simulink model "am"  (R2013b)
settings: Solver=ode45  StartTime=0.0  StopTime=10.0  RelTol=1e-3
undefined symbols (not defined in the file): fdesignblkfcn, gcbh
libraries: dspsrcs4 x1
settings Model: Creator=Nouri  LastModifiedBy=Ali

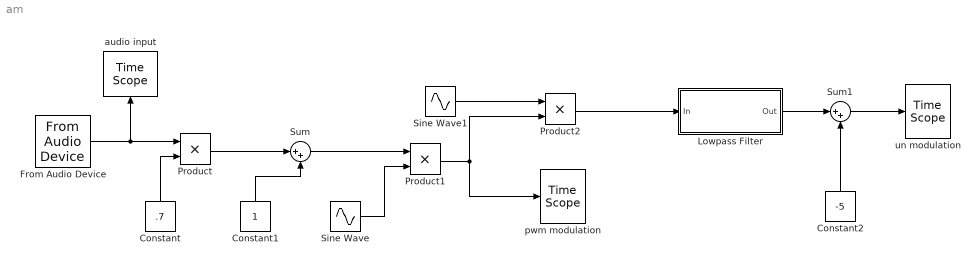
== system am ==
  Constant : Constant  Value=.7  OutDataTypeStr=single
  Constant1 : Constant  OutDataTypeStr=single
  Constant2 : Constant  Value=-5  OutDataTypeStr=single
  From Audio Device : dspsrcs4/From Audio Device  deviceName=Default  numChannels=1  sampleRate=1200  deviceDatatype=Determine from output data type  autoBufferSize=on  bufferSize=4096  queueDuration=5  frameSize=1  outputDatatype=single  defaultInputChannelMapping=on  inputChannelMapping=1:2
  Lowpass Filter : Subsystem  DialogController=fdesignblkfcn  InitFcn=fdesignblkfcn(gcbh, {'InitFcn'});  mask(Lowpass Filter){}
      mask help: Design a lowpass filter
      settings: CopyFcn=fdesignblkfcn(gcbh, {'CopyFcn'});
      mask Help: helpview(mapfilelocation('dsp'), 'dsplowpassfilter');
      mask Display: disp('Lowpass')
  Product : Product
  Product1 : Product
  Product2 : Product
  Sine Wave : Sin  Amplitude=2  Frequency=20000  SampleTime=0
  Sine Wave1 : Sin  Amplitude=2  Frequency=20000  SampleTime=0
  Sum : Sum  Inputs=|++
  Sum1 : Sum  Inputs=|++
  audio input : TimeScope  DefaultConfigurationName=spbscopes.TimeScopeBlockCfg
      settings: CopyFcn=scopeextensions.ScopeBlock.onCoreBlockCopy(gcbh);  DeleteFcn=scopeextensions.ScopeBlock.callback(gcbh, 'onBlockDelete');  PreSaveFcn=scopeextensions.ScopeBlock.callback(gcbh, 'onModelSave');  NameChangeFcn=scopeextensions.ScopeBlock.callback(gcbh, 'onBlockRename');  DestroyFcn=scopeextensions.ScopeBlock.onBlockDestroy(gcbh)  CloseFcn=scopeextensions.ScopeBlock.callback(gcbh, 'onBlockClose');  PreDeleteFcn=scopeextensions.ScopeBlock.callback(gcbh, 'onBlockPreDelete');
  pwm modulation : TimeScope  DefaultConfigurationName=spbscopes.TimeScopeBlockCfg
      settings: CopyFcn=scopeextensions.ScopeBlock.onCoreBlockCopy(gcbh);  DeleteFcn=scopeextensions.ScopeBlock.callback(gcbh, 'onBlockDelete');  PreSaveFcn=scopeextensions.ScopeBlock.callback(gcbh, 'onModelSave');  NameChangeFcn=scopeextensions.ScopeBlock.callback(gcbh, 'onBlockRename');  DestroyFcn=scopeextensions.ScopeBlock.onBlockDestroy(gcbh)  CloseFcn=scopeextensions.ScopeBlock.callback(gcbh, 'onBlockClose');  PreDeleteFcn=scopeextensions.ScopeBlock.callback(gcbh, 'onBlockPreDelete');
  un modulation : TimeScope  DefaultConfigurationName=spbscopes.TimeScopeBlockCfg
      settings: CopyFcn=scopeextensions.ScopeBlock.onCoreBlockCopy(gcbh);  DeleteFcn=scopeextensions.ScopeBlock.callback(gcbh, 'onBlockDelete');  PreSaveFcn=scopeextensions.ScopeBlock.callback(gcbh, 'onModelSave');  NameChangeFcn=scopeextensions.ScopeBlock.callback(gcbh, 'onBlockRename');  DestroyFcn=scopeextensions.ScopeBlock.onBlockDestroy(gcbh)  CloseFcn=scopeextensions.ScopeBlock.callback(gcbh, 'onBlockClose');  PreDeleteFcn=scopeextensions.ScopeBlock.callback(gcbh, 'onBlockPreDelete');
  wires:
  Constant/1 -> Product/2
  Product/1 -> Sum/1
  Sine Wave/1 -> Product1/2
  Product1/1 -> pwm modulation/1, Product2/2
  From Audio Device/1 -> audio input/1, Product/1
  Sum/1 -> Product1/1
  Sine Wave1/1 -> Product2/1
  Product2/1 -> Lowpass Filter/1(In)
  Lowpass Filter/1(Out) -> Sum1/1
  Sum1/1 -> un modulation/1
  Constant1/1 -> Sum/2
  Constant2/1 -> Sum1/2

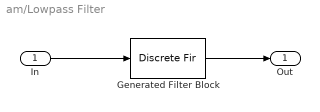
== system am/Lowpass Filter ==
  In : Inport
  Generated Filter Block : DiscreteFir  Tag=BlockMethodSubSystem  Coefficients=[-0.0024228738523270122 -0.0020832449820793308 0.0067703446401186241 0.016731945423488995 0.011117076081077605 -0.0062311454141444666 -0.0084016171860268225 0.0092567976151380314 0.012982883808855721 -0.010121234703278997 -0.018273518733782464 0.011431962071777964 0.026175888580407609 -0.012489027835322975 -0.037996623145463634 0.013388945199366932 0.05815546581472987 -0.014048043515808928 -0.10272466857882172 0.014462275771238403 0.31716649721769485 0.48538764678732516 0.31716649721769485 0.014462275771238403 -0.10272466857882172 -0.014048043515808928 0.05815546581472987 0.013388945199366932 -0.037996623145463634 -0.012489027835322975 0.026175888580407609 0.011431962071777964 -0.018273518733782464 -0.010121234703278997 0.012982883808855721 0.0092567976151380314 -0.0084016171860268225 -0.0062311454141444666 0.011117076081077605 0.016731945423488995 0.0067703446401186241 -0.0020832449820793308 -0.0024228738523270122]
  Out : Outport
  wires:
  In/1 -> Generated Filter Block/1
  Generated Filter Block/1 -> Out/1
